simulink model "wzorzec_final_ver"  (R2021b)
settings: Solver=ode5  StartTime=0.0  StopTime=Inf  FixedStep=0.01  RelTol=1e-3
undefined symbols (not defined in the file or in its folder): A, B, C, K, L, ur, xr
settings Model: SimulationMode=external  ExtModeTrigDuration=100000  Creator=STUDENT  LastModifiedBy=STUDENT
settings SolverCC: AlgebraicLoopSolver=TrustRegion  DecoupledContinuousIntegration=on  MinimalZcImpactIntegration=on
settings DataIOCC: ReturnWorkspaceOutputs=off
settings DebuggingCC: PregeneratedLibrarySubsystemCodeDiagnostic=none  SFMachineParentedDataDiag=warning  ArithmeticOperatorsInVariantConditions=warning
settings SFSimCC: SimUseLocalCustomCode=off  CustomCodeUndefinedFunction=UseInterfaceOnly
settings RTWCC: Description=Simulink Desktop Real-Time  SystemTargetFile=sldrt.tlc  TemplateMakefile=sldrt.tmf  RTWUseLocalCustomCode=off  RTWCompilerOptimization=on
settings CodeAppCC: MaxIdLength=95
settings SimulinkDesktopRealTimeCC: TargetPreCompLibLocation=C:\apps\MATLAB\R2021b\toolbox\sldrt\lib\win64

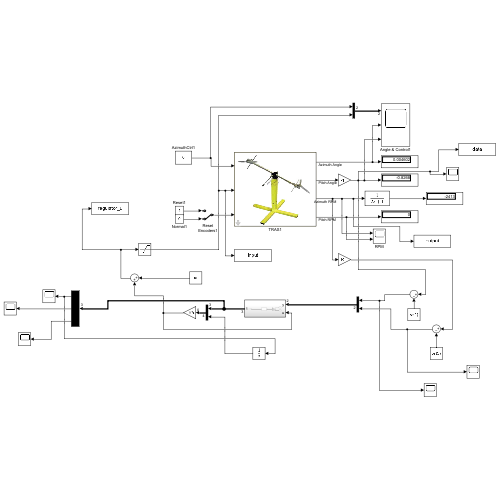
[thumbnail: Simulink's stored preview of the top-level diagram]
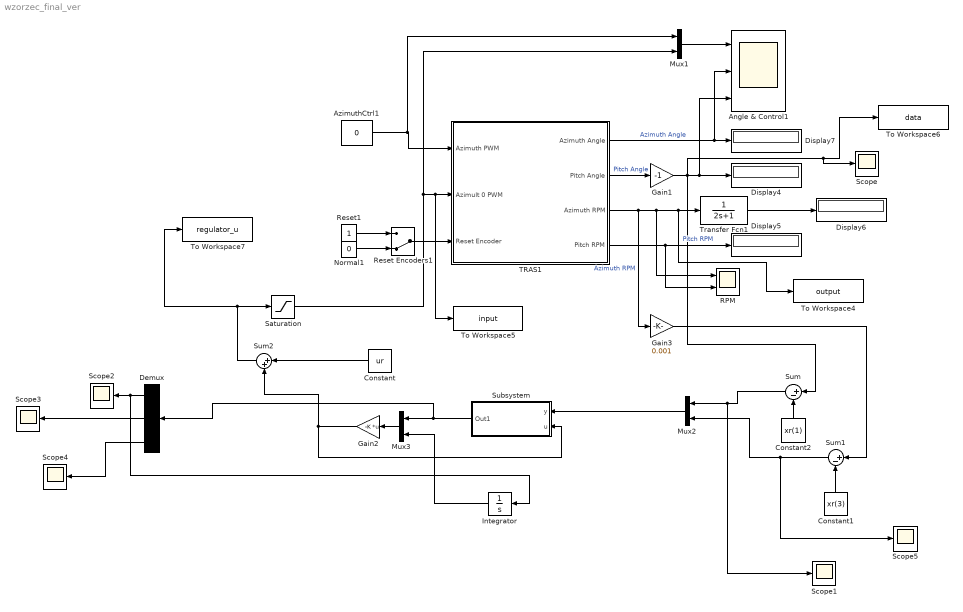
== system wzorzec_final_ver ==
  Angle & Control1 : Scope  NumInputPorts=3
  AzimuthCtrl1 : Constant  Value=0
  Constant : Constant  Value=ur
  Constant1 : Constant  Value=xr(3)
  Constant2 : Constant  Value=xr(1)
  Demux : Demux  Outputs=3
  Display{4..7} (4 alike) : Display
  Gain1 : Gain  Gain=-1
  Gain2 : Gain  Gain=-K  Multiplication=Matrix(K*u)
  Gain3 : Gain  Gain=0.001
  Integrator : Integrator
  Mux1 : Mux  Inputs=2
  Mux2 : Mux  Inputs=2
  Mux3 : Mux  Inputs=2
  Normal1 : Constant  Value=0
  RPM : Scope  NumInputPorts=2
  Reset Encoders1 : ManualSwitch  CurrentSetting=0
  Reset1 : Constant
  Saturation : Saturate  UpperLimit=0.6  LowerLimit=-0.6
  Scope{,1..5} (6 alike) : Scope
  Subsystem : Subsystem
  Sum : Sum  Inputs=|+-
  Sum1 : Sum  Inputs=|+-
  Sum2 : Sum  Inputs=|++
  TRAS1 : Subsystem  mask{BaseAddress=57088, T0=0.01}
      mask prompts: BaseAddress "Base Address:"; T0 "Sampling Period:"
      mask Display: image('TRAS.JPG')
  To Workspace4 : ToWorkspace  VariableName=output  SaveFormat=Structure With Time  SampleTime=0.01
  To Workspace5 : ToWorkspace  VariableName=input  SaveFormat=Structure With Time  SampleTime=0.01
  To Workspace6 : ToWorkspace  VariableName=data  SaveFormat=Structure With Time  SampleTime=0.01
  To Workspace7 : ToWorkspace  VariableName=regulator_u  SaveFormat=Structure With Time  SampleTime=-1
  Transfer Fcn1 : TransferFcn  Denominator=[2 1]
  wires:
  Gain2/1 -> Subsystem/2(u), Sum2/2
  Demux/1 -> Integrator/1, Scope2/1
  Demux/3 -> Scope4/1
  Subsystem/1(Out1) -> Demux/1, Mux3/1
  Sum/1 -> Scope1/1, Mux2/1
  Mux3/1 -> Gain2/1
  Saturation/1 -> Mux1/2, To Workspace5/1, TRAS1/2(Azimult 0 PWM)
  Constant/1 -> Sum2/1
  Mux1/1 -> Angle & Control1/1
  AzimuthCtrl1/1 -> Mux1/1, TRAS1/1(Azimuth PWM)
  Sum2/1 -> To Workspace7/1, Saturation/1
  Sum1/1 -> Scope5/1, Mux2/2
  Transfer Fcn1/1 -> Display6/1
  Demux/2 -> Scope3/1
  Constant1/1 -> Sum1/2
  TRAS1/4(Pitch RPM) -> RPM/2, Display5/1  "Pitch RPM"
  Reset1/1 -> Reset Encoders1/1
  TRAS1/3(Azimuth RPM) -> Gain3/1, To Workspace4/1, Transfer Fcn1/1, RPM/1  "Azimuth RPM"
  Constant2/1 -> Sum/2
  Normal1/1 -> Reset Encoders1/2
  TRAS1/1(Azimuth Angle) -> Angle & Control1/2, Display7/1  "Azimuth Angle"
  TRAS1/2(Pitch Angle) -> Gain1/1  "Pitch Angle"
  Reset Encoders1/1 -> TRAS1/3(Reset Encoder)
  Integrator/1 -> Mux3/2
  Gain1/1 -> Sum/1, Angle & Control1/3, Display4/1, Scope/1, To Workspace6/1
  Mux2/1 -> Subsystem/1(y)
  Gain3/1 -> Sum1/1

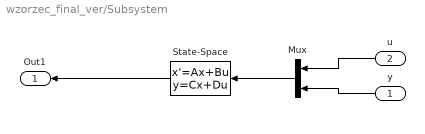
== system wzorzec_final_ver/Subsystem ==
  y : Inport
  u : Inport  Port=2
  Mux : Mux  Inputs=2
  State-Space : StateSpace  A=A-L*C  B=[B L]  C=eye(3)  D=zeros(3,3)  InitialCondition=zeros(3,1)
  Out1 : Outport
  wires:
  u/1 -> Mux/1
  y/1 -> Mux/2
  Mux/1 -> State-Space/1
  State-Space/1 -> Out1/1

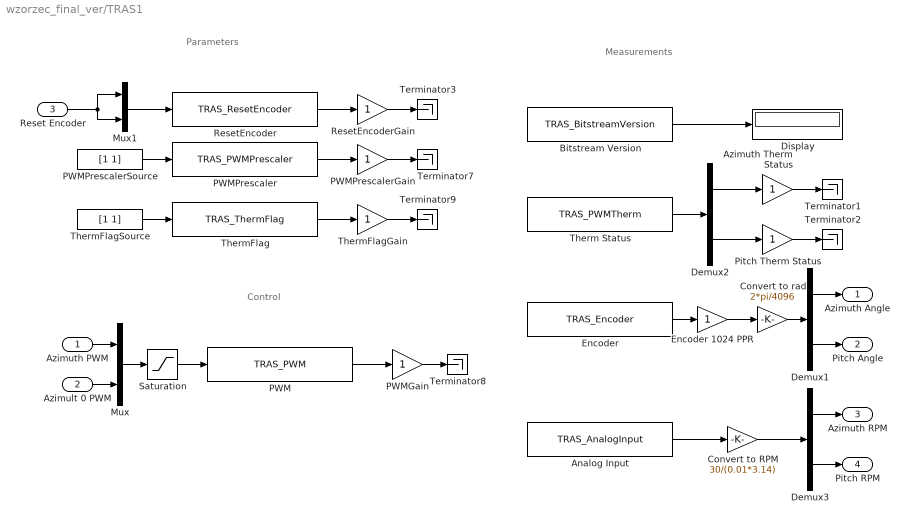
== system wzorzec_final_ver/TRAS1 ==
  note: Parameters
  note: Control
  note: Measurements
  Azimuth PWM : Inport
  Azimult 0 PWM : Inport  Port=2
  Reset Encoder : Inport  Port=3
  Analog Input : S-Function  FunctionName=TRAS_AnalogInput  Parameters=BaseAddress, [1 0], [1 1], T0  SFunctionDeploymentMode=off  EnableBusSupport=off
  Azimuth Therm Status : Gain  SaturateOnIntegerOverflow=on  OutDataTypeStr=Inherit: Same as input  ParamDataTypeStr=Inherit: Same as input
  Bitstream Version : S-Function  FunctionName=TRAS_BitstreamVersion  Parameters=BaseAddress, T0  SFunctionDeploymentMode=off  EnableBusSupport=off
  Convert to RPM : Gain  Gain=30/(0.01*3.14)  SaturateOnIntegerOverflow=on  OutDataTypeStr=Inherit: Same as input  ParamDataTypeStr=Inherit: Same as input
  Convert to rad : Gain  Gain=2*pi/4096  SaturateOnIntegerOverflow=on  OutDataTypeStr=Inherit: Same as input  ParamDataTypeStr=Inherit: Same as input
  Demux1 : Demux  Outputs=2
      settings: DisplayOption=none
  Demux2 : Demux  Outputs=2
      settings: DisplayOption=none
  Demux3 : Demux  Outputs=2
      settings: DisplayOption=none
  Display : Display
  Encoder : S-Function  FunctionName=TRAS_Encoder  Parameters=BaseAddress, T0  SFunctionDeploymentMode=off  EnableBusSupport=off
  Encoder 1024 PPR : Gain  SaturateOnIntegerOverflow=on  OutDataTypeStr=Inherit: Same as input  ParamDataTypeStr=Inherit: Same as input
  Mux : Mux  Inputs=2
  Mux1 : Mux  Inputs=2
  PWM : S-Function  FunctionName=TRAS_PWM  Parameters=BaseAddress, T0  SFunctionDeploymentMode=off  EnableBusSupport=off
  PWMGain : Gain  SaturateOnIntegerOverflow=on  OutDataTypeStr=Inherit: Same as input  ParamDataTypeStr=Inherit: Same as input
  PWMPrescaler : S-Function  FunctionName=TRAS_PWMPrescaler  Parameters=BaseAddress, T0  SFunctionDeploymentMode=off  EnableBusSupport=off
  PWMPrescalerGain : Gain  SaturateOnIntegerOverflow=on  OutDataTypeStr=Inherit: Same as input  ParamDataTypeStr=Inherit: Same as input
  PWMPrescalerSource : Constant  Value=[1 1]
  Pitch Therm Status : Gain  SaturateOnIntegerOverflow=on  OutDataTypeStr=Inherit: Same as input  ParamDataTypeStr=Inherit: Same as input
  ResetEncoder : S-Function  FunctionName=TRAS_ResetEncoder  Parameters=BaseAddress, T0  SFunctionDeploymentMode=off  EnableBusSupport=off
  ResetEncoderGain : Gain  SaturateOnIntegerOverflow=on  OutDataTypeStr=Inherit: Same as input  ParamDataTypeStr=Inherit: Same as input
  Saturation : Saturate  UpperLimit=1  LowerLimit=-1
  Terminator{1..3,7..9} (6 alike) : Terminator
  Therm Status : S-Function  FunctionName=TRAS_PWMTherm  Parameters=BaseAddress, T0  SFunctionDeploymentMode=off  EnableBusSupport=off
  "ThermFlag " : S-Function  FunctionName=TRAS_ThermFlag  Parameters=BaseAddress, T0  SFunctionDeploymentMode=off  EnableBusSupport=off
  ThermFlagGain : Gain  SaturateOnIntegerOverflow=on  OutDataTypeStr=Inherit: Same as input  ParamDataTypeStr=Inherit: Same as input
  ThermFlagSource : Constant  Value=[1 1]
  Azimuth Angle : Outport  VectorParamsAs1DForOutWhenUnconnected=off
  Pitch Angle : Outport  Port=2  VectorParamsAs1DForOutWhenUnconnected=off
  Azimuth RPM : Outport  Port=3  VectorParamsAs1DForOutWhenUnconnected=off
  Pitch RPM : Outport  Port=4  VectorParamsAs1DForOutWhenUnconnected=off
  wires:
  Encoder 1024 PPR/1 -> Convert to rad/1
  Encoder/1 -> Encoder 1024 PPR/1
  Saturation/1 -> PWM/1
  Mux/1 -> Saturation/1
  PWM/1 -> PWMGain/1
  PWMGain/1 -> Terminator8/1
  ResetEncoder/1 -> ResetEncoderGain/1
  PWMPrescaler/1 -> PWMPrescalerGain/1
  Mux1/1 -> ResetEncoder/1
  PWMPrescalerSource/1 -> PWMPrescaler/1
  ResetEncoderGain/1 -> Terminator3/1
  PWMPrescalerGain/1 -> Terminator7/1
  Azimult 0 PWM/1 -> Mux/2
  Azimuth PWM/1 -> Mux/1
  Demux1/2 -> Pitch Angle/1
  Convert to rad/1 -> Demux1/1
  Demux1/1 -> Azimuth Angle/1
  Therm Status/1 -> Demux2/1
  Demux2/2 -> Pitch Therm Status/1
  Demux2/1 -> Azimuth Therm Status/1
  Azimuth Therm Status/1 -> Terminator1/1
  Pitch Therm Status/1 -> Terminator2/1
  Bitstream Version/1 -> Display/1
  Analog Input/1 -> Convert to RPM/1
  Demux3/2 -> Pitch RPM/1
  Demux3/1 -> Azimuth RPM/1
  Reset Encoder/1 -> Mux1/1, Mux1/2
  Convert to RPM/1 -> Demux3/1
  "ThermFlag "/1 -> ThermFlagGain/1
  ThermFlagSource/1 -> "ThermFlag "/1
  ThermFlagGain/1 -> Terminator9/1
